simulink model "yxf_RLC"  (R2022b)
settings: Solver=VariableStepAuto  StartTime=0.0  StopTime=10.0  RelTol=1e-3
settings Model: Creator=11217  LastModifiedBy=11217

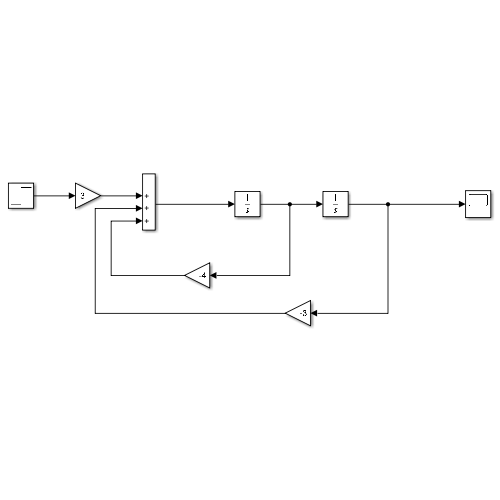
[thumbnail: Simulink's stored preview of the top-level diagram]
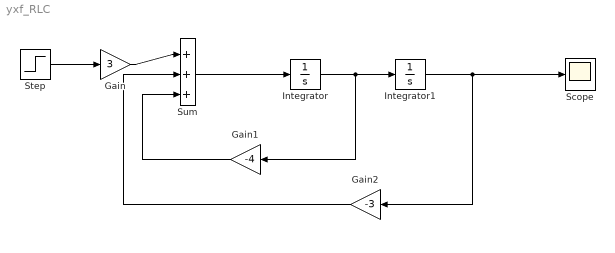
== system yxf_RLC ==
  Gain : Gain  Gain=3
  Gain1 : Gain  Gain=-4
  Gain2 : Gain  Gain=-3
  Integrator : Integrator
  Integrator1 : Integrator  InitialCondition=0.5
  Scope : Scope
  Step : Step  SampleTime=0
  Sum : Sum  Inputs=|+++
  wires:
  Step/1 -> Gain/1
  Gain/1 -> Sum/1
  Sum/1 -> Integrator/1
  Integrator/1 -> Gain1/1, Integrator1/1
  Integrator1/1 -> Scope/1, Gain2/1
  Gain2/1 -> Sum/2
  Gain1/1 -> Sum/3
